simulink model "WormAndGearConstraintMain"  (R2024a)
settings: Solver=ode45  StartTime=0.0  StopTime=120  MaxStep=0.01  RelTol=1e-3
PreLoadFcn:
  | addpath(fullfile('WormAndGearConstraintSupport','Data'));
  | addpath(fullfile('WormAndGearConstraintSupport','Scripts'));
model workspace: external: MATLAB File WormAndGearConstraintParameters.m (data not in the file)
undefined symbols (not defined in the file or in its folder): slewdrive, X, Y, Z
libraries: sm_lib x75, nesl_utility x38, fl_lib x32, WormAndGearConstraintLibrary x24, neural x20, ee_lib x6, slpidlib x6, fl_ps_legacy_lib x1
(part 5 of 5)

== system WormAndGearConstraintMain/Solar Array/Solar Tracker2/Slew Drive1/Worm and Gear Assembly/Gear ==
  Bottom : sm_lib/Body Elements/Extruded Solid  ExtrusionType=General  PolygonNumSides=3  PolygonOuterRadius=1  PolygonOuterRadiusUnits=m  ExportEntireGeometry=off  ExtrusionCrossSection=botCrossSection  ExtrusionCrossSectionUnits=m  ExportConvexHullGeometry=off  ExtrusionLength=length  ExtrusionLengthUnits=m  InertiaType=CalculateFromGeometry  BasedOnType=Density  Density=rho  DensityUnits=kg/m^3  Mass=1  MassUnits=kg  CenterOfMass=[0 0 0]  CenterOfMassUnits=m  MomentsOfInertia=[1 1 1]  MomentsOfInertiaUnits=kg*m^2  ProductsOfInertia=[1 1 1]  ProductsOfInertiaUnits=kg*m^2  GraphicType=FromGeometry  MarkerShape=Sphere  MarkerSize=10  GraphicVisPropType=SimpleVisualProperties  GraphicDiffuseColor=sliceColor  GraphicOpacity=1.0  GraphicSpecularColor=[0.5 0.5 0.5 1.0]  GraphicAmbientColor=[0.15 0.15 0.15 1.0]  GraphicEmissiveColor=[0.0 0.0 0.0 1.0]  GraphicShininess=75  DoExposeReferenceFrame=on  SerializedFrames=<Frames/>
  Left : sm_lib/Body Elements/Extruded Solid  ExtrusionType=General  PolygonNumSides=3  PolygonOuterRadius=1  PolygonOuterRadiusUnits=m  ExportEntireGeometry=off  ExtrusionCrossSection=leftCrossSection  ExtrusionCrossSectionUnits=m  ExportConvexHullGeometry=off  ExtrusionLength=length  ExtrusionLengthUnits=m  InertiaType=CalculateFromGeometry  BasedOnType=Density  Density=rho  DensityUnits=kg/m^3  Mass=1  MassUnits=kg  CenterOfMass=[0 0 0]  CenterOfMassUnits=m  MomentsOfInertia=[1 1 1]  MomentsOfInertiaUnits=kg*m^2  ProductsOfInertia=[1 1 1]  ProductsOfInertiaUnits=kg*m^2  GraphicType=FromGeometry  MarkerShape=Sphere  MarkerSize=10  GraphicVisPropType=SimpleVisualProperties  GraphicDiffuseColor=mainColor  GraphicOpacity=1.0  GraphicSpecularColor=[0.5 0.5 0.5 1.0]  GraphicAmbientColor=[0.15 0.15 0.15 1.0]  GraphicEmissiveColor=[0.0 0.0 0.0 1.0]  GraphicShininess=75  DoExposeReferenceFrame=on  SerializedFrames=<Frames/>
  Left End xForm : sm_lib/Frames and Transforms/Rigid Transform  RotationMethod=None  FollAlignAxisA=+X  BaseAlignAxisA=+Y  FollAlignAxisB=+Y  BaseAlignAxisB=+Z  RotationStandardAxis=+Z  RotationAngle=0.0  RotationAngleUnits=deg  RotationArbitraryAxis=[0 0 1]  RotationSequenceAxes=FollowerAxes  RotationSequence=XYX  RotationSequenceAngles=[0 0 0]  RotationSequenceAnglesUnits=deg  RotationMatrix=[1 0 0; 0 1 0; 0 0 1]  Quaternion=[1 0 0 0]  TranslationMethod=StandardAxis  TranslationCartesianOffset=[0 0 0]  TranslationCartesianOffsetUnits=m  TranslationStandardAxis=-Z  TranslationStandardOffset=0.5*length  TranslationStandardOffsetUnits=m  TranslationROffset=0  TranslationROffsetUnits=m  TranslationThetaOffset=0  TranslationThetaOffsetUnits=deg  TranslationZOffset=0  TranslationZOffsetUnits=m
  Right : sm_lib/Body Elements/Extruded Solid  ExtrusionType=General  PolygonNumSides=3  PolygonOuterRadius=1  PolygonOuterRadiusUnits=m  ExportEntireGeometry=off  ExtrusionCrossSection=rightCrossSection  ExtrusionCrossSectionUnits=m  ExportConvexHullGeometry=off  ExtrusionLength=length  ExtrusionLengthUnits=m  InertiaType=CalculateFromGeometry  BasedOnType=Density  Density=rho  DensityUnits=kg/m^3  Mass=1  MassUnits=kg  CenterOfMass=[0 0 0]  CenterOfMassUnits=m  MomentsOfInertia=[1 1 1]  MomentsOfInertiaUnits=kg*m^2  ProductsOfInertia=[1 1 1]  ProductsOfInertiaUnits=kg*m^2  GraphicType=FromGeometry  MarkerShape=Sphere  MarkerSize=10  GraphicVisPropType=SimpleVisualProperties  GraphicDiffuseColor=mainColor  GraphicOpacity=1.0  GraphicSpecularColor=[0.5 0.5 0.5 1.0]  GraphicAmbientColor=[0.15 0.15 0.15 1.0]  GraphicEmissiveColor=[0.0 0.0 0.0 1.0]  GraphicShininess=75  DoExposeReferenceFrame=on  SerializedFrames=<Frames/>
  Right End xForm : sm_lib/Frames and Transforms/Rigid Transform  RotationMethod=None  FollAlignAxisA=+X  BaseAlignAxisA=+Y  FollAlignAxisB=+Y  BaseAlignAxisB=+Z  RotationStandardAxis=+Z  RotationAngle=0.0  RotationAngleUnits=deg  RotationArbitraryAxis=[0 0 1]  RotationSequenceAxes=FollowerAxes  RotationSequence=XYX  RotationSequenceAngles=[0 0 0]  RotationSequenceAnglesUnits=deg  RotationMatrix=[1 0 0; 0 1 0; 0 0 1]  Quaternion=[1 0 0 0]  TranslationMethod=StandardAxis  TranslationCartesianOffset=[0 0 0]  TranslationCartesianOffsetUnits=m  TranslationStandardAxis=+Z  TranslationStandardOffset=0.5*length  TranslationStandardOffsetUnits=m  TranslationROffset=0  TranslationROffsetUnits=m  TranslationThetaOffset=0  TranslationThetaOffsetUnits=deg  TranslationZOffset=0  TranslationZOffsetUnits=m
  Top : sm_lib/Body Elements/Extruded Solid  ExtrusionType=General  PolygonNumSides=3  PolygonOuterRadius=1  PolygonOuterRadiusUnits=m  ExportEntireGeometry=off  ExtrusionCrossSection=topCrossSection  ExtrusionCrossSectionUnits=m  ExportConvexHullGeometry=off  ExtrusionLength=length  ExtrusionLengthUnits=m  InertiaType=CalculateFromGeometry  BasedOnType=Density  Density=rho  DensityUnits=kg/m^3  Mass=1  MassUnits=kg  CenterOfMass=[0 0 0]  CenterOfMassUnits=m  MomentsOfInertia=[1 1 1]  MomentsOfInertiaUnits=kg*m^2  ProductsOfInertia=[1 1 1]  ProductsOfInertiaUnits=kg*m^2  GraphicType=FromGeometry  MarkerShape=Sphere  MarkerSize=10  GraphicVisPropType=SimpleVisualProperties  GraphicDiffuseColor=sliceColor  GraphicOpacity=1.0  GraphicSpecularColor=[0.5 0.5 0.5 1.0]  GraphicAmbientColor=[0.15 0.15 0.15 1.0]  GraphicEmissiveColor=[0.0 0.0 0.0 1.0]  GraphicShininess=75  DoExposeReferenceFrame=on  SerializedFrames=<Frames/>
  L : PMIOPort  Side=Left
  R : PMIOPort  Port=2  Side=Right
  connections:
  L/RConn1 -- Left End xForm/RConn1
  Top/RConn1 -- Bottom/RConn1 -- Right/RConn1 -- Right End xForm/LConn1 -- Left End xForm/LConn1 -- Left/RConn1
  R/RConn1 -- Right End xForm/RConn1

== system WormAndGearConstraintMain/Solar Array/Solar Tracker2/Slew Drive1/Worm and Gear Assembly/Worm ==
  Left Non-Threaded : WormAndGearConstraintLibrary/Sliced Hollow Cylinder  outerRadius=wormNonThreadedRadius  thickness=wormNonThreadedThickness  length=wormNonThreadedLength  sliceThickness=wormSliceProportion*wormNonThreadedRadius  rho=wormRho  mainColor=wormColor  sliceColor=wormSliceColor
  Right Non-Threaded : WormAndGearConstraintLibrary/Sliced Hollow Cylinder  outerRadius=wormNonThreadedRadius  thickness=wormNonThreadedThickness  length=wormNonThreadedLength  sliceThickness=wormSliceProportion*wormNonThreadedRadius  rho=wormRho  mainColor=wormColor  sliceColor=wormSliceColor
  Threaded : WormAndGearConstraintLibrary/Sliced Hollow Cylinder  outerRadius=wormRadius  thickness=wormThreadedThickness  length=wormThreadedLength  sliceThickness=wormSliceProportion*wormRadius  rho=wormRho  mainColor=wormColor  sliceColor=wormSliceColor
  L : PMIOPort  Side=Left
  R : PMIOPort  Port=2  Side=Right
  connections:
  Threaded/LConn1 -- Left Non-Threaded/RConn1
  Threaded/RConn1 -- Right Non-Threaded/LConn1
  R/RConn1 -- Right Non-Threaded/RConn1
  Left Non-Threaded/LConn1 -- L/RConn1

== system WormAndGearConstraintMain/Solar Array/Solar Tracker3/Slew Drive/Worm and Gear Assembly/Gear ==
  Bottom : sm_lib/Body Elements/Extruded Solid  ExtrusionType=General  PolygonNumSides=3  PolygonOuterRadius=1  PolygonOuterRadiusUnits=m  ExportEntireGeometry=off  ExtrusionCrossSection=botCrossSection  ExtrusionCrossSectionUnits=m  ExportConvexHullGeometry=off  ExtrusionLength=length  ExtrusionLengthUnits=m  InertiaType=CalculateFromGeometry  BasedOnType=Density  Density=rho  DensityUnits=kg/m^3  Mass=1  MassUnits=kg  CenterOfMass=[0 0 0]  CenterOfMassUnits=m  MomentsOfInertia=[1 1 1]  MomentsOfInertiaUnits=kg*m^2  ProductsOfInertia=[1 1 1]  ProductsOfInertiaUnits=kg*m^2  GraphicType=FromGeometry  MarkerShape=Sphere  MarkerSize=10  GraphicVisPropType=SimpleVisualProperties  GraphicDiffuseColor=sliceColor  GraphicOpacity=1.0  GraphicSpecularColor=[0.5 0.5 0.5 1.0]  GraphicAmbientColor=[0.15 0.15 0.15 1.0]  GraphicEmissiveColor=[0.0 0.0 0.0 1.0]  GraphicShininess=75  DoExposeReferenceFrame=on  SerializedFrames=<Frames/>
  Left : sm_lib/Body Elements/Extruded Solid  ExtrusionType=General  PolygonNumSides=3  PolygonOuterRadius=1  PolygonOuterRadiusUnits=m  ExportEntireGeometry=off  ExtrusionCrossSection=leftCrossSection  ExtrusionCrossSectionUnits=m  ExportConvexHullGeometry=off  ExtrusionLength=length  ExtrusionLengthUnits=m  InertiaType=CalculateFromGeometry  BasedOnType=Density  Density=rho  DensityUnits=kg/m^3  Mass=1  MassUnits=kg  CenterOfMass=[0 0 0]  CenterOfMassUnits=m  MomentsOfInertia=[1 1 1]  MomentsOfInertiaUnits=kg*m^2  ProductsOfInertia=[1 1 1]  ProductsOfInertiaUnits=kg*m^2  GraphicType=FromGeometry  MarkerShape=Sphere  MarkerSize=10  GraphicVisPropType=SimpleVisualProperties  GraphicDiffuseColor=mainColor  GraphicOpacity=1.0  GraphicSpecularColor=[0.5 0.5 0.5 1.0]  GraphicAmbientColor=[0.15 0.15 0.15 1.0]  GraphicEmissiveColor=[0.0 0.0 0.0 1.0]  GraphicShininess=75  DoExposeReferenceFrame=on  SerializedFrames=<Frames/>
  Left End xForm : sm_lib/Frames and Transforms/Rigid Transform  RotationMethod=None  FollAlignAxisA=+X  BaseAlignAxisA=+Y  FollAlignAxisB=+Y  BaseAlignAxisB=+Z  RotationStandardAxis=+Z  RotationAngle=0.0  RotationAngleUnits=deg  RotationArbitraryAxis=[0 0 1]  RotationSequenceAxes=FollowerAxes  RotationSequence=XYX  RotationSequenceAngles=[0 0 0]  RotationSequenceAnglesUnits=deg  RotationMatrix=[1 0 0; 0 1 0; 0 0 1]  Quaternion=[1 0 0 0]  TranslationMethod=StandardAxis  TranslationCartesianOffset=[0 0 0]  TranslationCartesianOffsetUnits=m  TranslationStandardAxis=-Z  TranslationStandardOffset=0.5*length  TranslationStandardOffsetUnits=m  TranslationROffset=0  TranslationROffsetUnits=m  TranslationThetaOffset=0  TranslationThetaOffsetUnits=deg  TranslationZOffset=0  TranslationZOffsetUnits=m
  Right : sm_lib/Body Elements/Extruded Solid  ExtrusionType=General  PolygonNumSides=3  PolygonOuterRadius=1  PolygonOuterRadiusUnits=m  ExportEntireGeometry=off  ExtrusionCrossSection=rightCrossSection  ExtrusionCrossSectionUnits=m  ExportConvexHullGeometry=off  ExtrusionLength=length  ExtrusionLengthUnits=m  InertiaType=CalculateFromGeometry  BasedOnType=Density  Density=rho  DensityUnits=kg/m^3  Mass=1  MassUnits=kg  CenterOfMass=[0 0 0]  CenterOfMassUnits=m  MomentsOfInertia=[1 1 1]  MomentsOfInertiaUnits=kg*m^2  ProductsOfInertia=[1 1 1]  ProductsOfInertiaUnits=kg*m^2  GraphicType=FromGeometry  MarkerShape=Sphere  MarkerSize=10  GraphicVisPropType=SimpleVisualProperties  GraphicDiffuseColor=mainColor  GraphicOpacity=1.0  GraphicSpecularColor=[0.5 0.5 0.5 1.0]  GraphicAmbientColor=[0.15 0.15 0.15 1.0]  GraphicEmissiveColor=[0.0 0.0 0.0 1.0]  GraphicShininess=75  DoExposeReferenceFrame=on  SerializedFrames=<Frames/>
  Right End xForm : sm_lib/Frames and Transforms/Rigid Transform  RotationMethod=None  FollAlignAxisA=+X  BaseAlignAxisA=+Y  FollAlignAxisB=+Y  BaseAlignAxisB=+Z  RotationStandardAxis=+Z  RotationAngle=0.0  RotationAngleUnits=deg  RotationArbitraryAxis=[0 0 1]  RotationSequenceAxes=FollowerAxes  RotationSequence=XYX  RotationSequenceAngles=[0 0 0]  RotationSequenceAnglesUnits=deg  RotationMatrix=[1 0 0; 0 1 0; 0 0 1]  Quaternion=[1 0 0 0]  TranslationMethod=StandardAxis  TranslationCartesianOffset=[0 0 0]  TranslationCartesianOffsetUnits=m  TranslationStandardAxis=+Z  TranslationStandardOffset=0.5*length  TranslationStandardOffsetUnits=m  TranslationROffset=0  TranslationROffsetUnits=m  TranslationThetaOffset=0  TranslationThetaOffsetUnits=deg  TranslationZOffset=0  TranslationZOffsetUnits=m
  Top : sm_lib/Body Elements/Extruded Solid  ExtrusionType=General  PolygonNumSides=3  PolygonOuterRadius=1  PolygonOuterRadiusUnits=m  ExportEntireGeometry=off  ExtrusionCrossSection=topCrossSection  ExtrusionCrossSectionUnits=m  ExportConvexHullGeometry=off  ExtrusionLength=length  ExtrusionLengthUnits=m  InertiaType=CalculateFromGeometry  BasedOnType=Density  Density=rho  DensityUnits=kg/m^3  Mass=1  MassUnits=kg  CenterOfMass=[0 0 0]  CenterOfMassUnits=m  MomentsOfInertia=[1 1 1]  MomentsOfInertiaUnits=kg*m^2  ProductsOfInertia=[1 1 1]  ProductsOfInertiaUnits=kg*m^2  GraphicType=FromGeometry  MarkerShape=Sphere  MarkerSize=10  GraphicVisPropType=SimpleVisualProperties  GraphicDiffuseColor=sliceColor  GraphicOpacity=1.0  GraphicSpecularColor=[0.5 0.5 0.5 1.0]  GraphicAmbientColor=[0.15 0.15 0.15 1.0]  GraphicEmissiveColor=[0.0 0.0 0.0 1.0]  GraphicShininess=75  DoExposeReferenceFrame=on  SerializedFrames=<Frames/>
  L : PMIOPort  Side=Left
  R : PMIOPort  Port=2  Side=Right
  connections:
  L/RConn1 -- Left End xForm/RConn1
  Top/RConn1 -- Bottom/RConn1 -- Right/RConn1 -- Right End xForm/LConn1 -- Left End xForm/LConn1 -- Left/RConn1
  R/RConn1 -- Right End xForm/RConn1

== system WormAndGearConstraintMain/Solar Array/Solar Tracker3/Slew Drive/Worm and Gear Assembly/Worm ==
  Left Non-Threaded : WormAndGearConstraintLibrary/Sliced Hollow Cylinder  outerRadius=wormNonThreadedRadius  thickness=wormNonThreadedThickness  length=wormNonThreadedLength  sliceThickness=wormSliceProportion*wormNonThreadedRadius  rho=wormRho  mainColor=wormColor  sliceColor=wormSliceColor
  Right Non-Threaded : WormAndGearConstraintLibrary/Sliced Hollow Cylinder  outerRadius=wormNonThreadedRadius  thickness=wormNonThreadedThickness  length=wormNonThreadedLength  sliceThickness=wormSliceProportion*wormNonThreadedRadius  rho=wormRho  mainColor=wormColor  sliceColor=wormSliceColor
  Threaded : WormAndGearConstraintLibrary/Sliced Hollow Cylinder  outerRadius=wormRadius  thickness=wormThreadedThickness  length=wormThreadedLength  sliceThickness=wormSliceProportion*wormRadius  rho=wormRho  mainColor=wormColor  sliceColor=wormSliceColor
  L : PMIOPort  Side=Left
  R : PMIOPort  Port=2  Side=Right
  connections:
  Threaded/LConn1 -- Left Non-Threaded/RConn1
  Threaded/RConn1 -- Right Non-Threaded/LConn1
  R/RConn1 -- Right Non-Threaded/RConn1
  Left Non-Threaded/LConn1 -- L/RConn1

== matlab function WormAndGearConstraintMain/Solar Array/MATLAB Function ==
  data: lat input; output output; lon input
function output = generateInput(lat, lon)
    % Get the current date and time
    datetimeNow = datetime('now');
    [~, month, day , hour, ~, ~] = datevec(datetimeNow);

    % Create the output array
    output = [lat; lon; month; day; hour];
end

== matlab function WormAndGearConstraintMain/MATLAB Function ==
  data latitude settings: description=Year input
  data: latitude input double size=1; azimuth output size=1; longitude input double size=1; timeVector input double size=[1 6]; elevation output double size=1
function [azimuth, elevation] = calculateSolarPosition(latitude, longitude, timeVector)
    year = timeVector(1);
    month = timeVector(2);
    day = timeVector(3);
    hour = timeVector(4);
    minute = timeVector(5);
    second = timeVector(6);

    % Calculate Julian Date
    JD = calculateJulianDate(year, month, day, hour, minute, second);
    
    % Calculate days since J2000.0
    n = daysSinceJ2000(JD);
    
    % Calculate mean longitude of the sun
    L = meanLongitudeSun(n);
    
    % Calculate mean anomaly of the sun
    g = meanAnomalySun(n);
    
    % Calculate ecliptic longitude of the sun
    lambda = eclipticLongitudeSun(L, g);
    
    % Calculate obliquity of the ecliptic
    epsilon = obliquityEcliptic(n);
    
    % Calculate right ascension and declination of the sun
    [alpha, delta] = rightAscensionDeclination(lambda, epsilon);
    
    % Calculate local sidereal time
    LST = localSiderealTime(n, longitude, hour, minute, second);
    
    % Calculate hour angle
    H = hourAngle(LST, alpha);
    
    % Calculate elevation and azimuth angles
    [elevation, azimuth] = solarElevationAzimuth(latitude, delta, H);
end

% Helper functions
function JD = calculateJulianDate(year, month, day, hour, minute, second)
    if month <= 2
        year = year - 1;
        month = month + 12;
    end
    A = floor(year / 100);
    B = 2 - A + floor(A / 4);
    JD = floor(365.25 * (year + 4716)) + floor(30.6001 * (month + 1)) + day + B - 1524.5 ...
        + (hour + minute / 60 + second / 3600) / 24;
end

function n = daysSinceJ2000(JD)
    JD_J2000 = 2451545.0;  % Julian Date of J2000.0
    n = JD - JD_J2000;
end

function L = meanLongitudeSun(n)
    L = mod(280.460 + 0.9856474 * n, 360);
end

function g = meanAnomalySun(n)
    g = mod(357.528 + 0.9856003 * n, 360);
end

function lambda = eclipticLongitudeSun(L, g)
    lambda = mod(L + 1.915 * sind(g) + 0.020 * sind(2 * g), 360);
end

function epsilon = obliquityEcliptic(n)
    epsilon = 23.439 - 0.0000004 * n;
end

function [alpha, delta] = rightAscensionDeclination(lambda, epsilon)
    alpha = atan2d(cosd(epsilon) * sind(lambda), cosd(lambda));
    delta = asind(sind(epsilon) * sind(lambda));
end

function LST = localSiderealTime(n, longitude, hour, minute, second)
    GMST = mod(6.697374558 + 0.06570982441908 * n + (hour + minute / 60 + second / 3600) * 1.00273790935, 24);
    LST = mod(GMST * 15 + longitude, 360);
end

function H = hourAngle(LST, alpha)
    H = mod(LST - alpha, 360);
end

function [elevation, azimuth] = solarElevationAzimuth(latitude, delta, H)
    elevation = asind(sind(latitude) * sind(delta) + cosd(latitude) * cosd(delta) * cosd(H));
    azimuth = atan2d(-sind(H), cosd(H) * sind(latitude) - tand(delta) * cosd(latitude));
    if azimuth < 0
        azimuth = azimuth + 360;
    end
end

== stateflow chart WormAndGearConstraintMain/Solar Array/stateflow logic chart ==
  state Night_time
    during:
    pitch_upd = 0 ;
    yaw_upd = 0 ;
  state Cloudy
    entry:
    hold_pitch = pitch ;
    hold_yaw  = yaw ;
    during :
    pitch_upd = hold_pitch
    yaw_upd = hold_yaw;
    exit:
    pitch_upd = hold_pitch
    yaw_upd = hold_yaw;
  state Daytime
    during :
    pitch_upd = pitch;
    yaw_upd = yaw;
  Cloudy -> Night_time [order 2] : [abs(pitch) > 1.48353]
  Night_time -> Cloudy [order 1] : [ irradiance <450 && abs(pitch)<=1.48353 ]
  Night_time -> Daytime [order 2] : [abs(pitch)<=1.48353]
  Daytime -> Night_time [order 1] : [abs(pitch) > 1.48353]
  (default) -> Daytime
  Daytime -> Cloudy [order 2] : [ irradiance < 450 ]
  Cloudy -> Daytime [order 1] : [abs(pitch)<=1.48353 && irradiance>= 450]
  data: yaw input; yaw_upd output; pitch input; pitch_upd output; hold_yaw local double size=1; hold_pitch local double size=1; irradiance input

== matlab function WormAndGearConstraintMain/MATLAB Function1 ==
  data: unused input double size=1; timeVector output double size=[1 6]
function timeVector = extractTimeFromClock(~)
    datetimeNow = datetime('now');
    [year, month, day, hour, minute, second] = datevec(datetimeNow);
    timeVector = [year, month, day, hour, minute, second];
end
